simulink model "Simulation_FL_BB"  (R2023a)
settings: Solver=VariableStepAuto  StartTime=0.0  StopTime=50  RelTol=1e-3
settings Model: Creator=j.acevedom  LastModifiedBy=j.acevedom

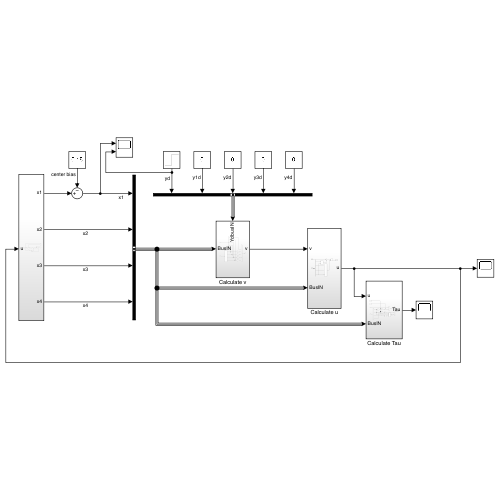
[thumbnail: Simulink's stored preview of the top-level diagram]
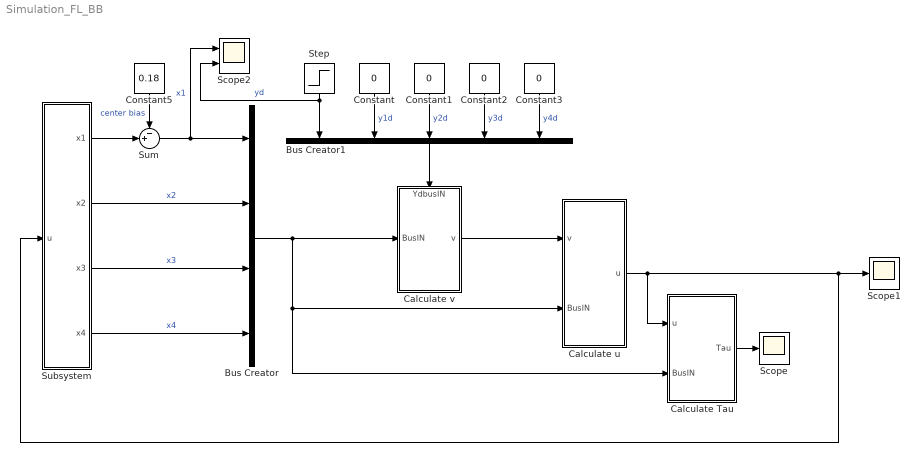
== system Simulation_FL_BB ==
  Bus Creator : BusCreator  Inputs=4
  Bus Creator1 : BusCreator  Inputs=5
  Calculate Tau : Subsystem
  Calculate u : Subsystem
  Calculate v : Subsystem
      settings: PortSchema="{\"entries\":[{\"content\":{\"sides\":[{\"content\":{\"connectorIds\":[\"In1\"]},\"type\":\"ConnectorPlacement.EquallySpacedRectSide\",\"uuid\":\"7c28e410-4806-4a94-8ccf-a14e347b0b8c\"},{\"content\":{\"connectorIds\":[\"Out1\"],\"side\":\"RIGHT\"},\"type\":\"ConnectorPlacement.EquallySpacedRectSide\",\"uuid\":\"f53d7206-bd2e-4f71-94df-5fcac3ff5314\"},{\"content\":{\"connectorIds\":[\"In2\"],\"side\":\"TOP\"},\"type\":\"ConnectorPlacement.EquallySpacedRectSide\",\"uuid\":\"6da5d2a6-a8d3-48a8-94f9-21942db04e1c\"}]},\"type\":\"ConnectorPlacement.EquallySpacedConnector\",\"uuid\":\"b4263dcd-b19e-4751-b906-56e55f698d2c\"}],\"packageUris\":[\"http://schema.mathworks.com/mf0/Connector/R2020b\"],\"version\":\"1.0\"}"
  Constant{,1..3} (4 alike) : Constant  Value=0
  Constant5 : Constant  Value=0.18
  Scope : Scope
  Scope1 : Scope
  Scope2 : Scope  NumInputPorts=2
  Step : Step  Time=10  After=0.1  SampleTime=0
  Subsystem : Subsystem
  Sum : Sum  Inputs=-+|
  wires:
  Calculate u/1(u) -> Scope1/1, Subsystem/1(u), Calculate Tau/1(u)
  Subsystem/3(x3) -> Bus Creator/3  "x3"
  Subsystem/4(x4) -> Bus Creator/4  "x4"
  Bus Creator/1 -> Calculate u/2(BusIN), Calculate Tau/2(BusIN), Calculate v/1(BusIN)
  Calculate v/1(v) -> Calculate u/1(v)
  Step/1 -> Scope2/2, Bus Creator1/1  "yd"
  Constant/1 -> Bus Creator1/2  "y1d"
  Constant1/1 -> Bus Creator1/3  "y2d"
  Constant2/1 -> Bus Creator1/4  "y3d"
  Constant3/1 -> Bus Creator1/5  "y4d"
  Bus Creator1/1 -> Calculate v/2(YdbusIN)
  Sum/1 -> Bus Creator/1, Scope2/1  "x1"
  Constant5/1 -> Sum/1  "center bias"
  Subsystem/2(x2) -> Bus Creator/2  "x2"
  Subsystem/1(x1) -> Sum/2
  Calculate Tau/1(Tau) -> Scope/1

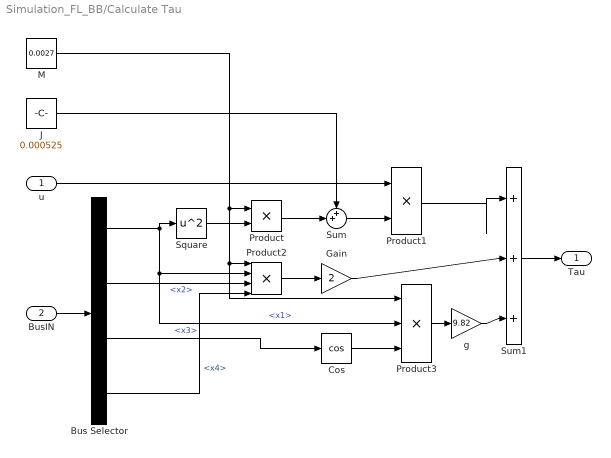
== system Simulation_FL_BB/Calculate Tau ==
  u : Inport
  BusIN : Inport  Port=2
  Bus Selector : BusSelector  OutputSignals=x1,x2,x3,x4
  Cos : Trigonometry  Operator=cos
  Gain : Gain  Gain=2
  J : Constant  Value=0.000525
  M : Constant  Value=0.0027
  Product : Product
  Product1 : Product
  Product2 : Product  Inputs=4
  Product3 : Product  Inputs=3
  Square : Math  Operator=square
  Sum : Sum  Inputs=++|
  Sum1 : Sum  Inputs=|+++
  g : Gain  Gain=9.82
  Tau : Outport
  wires:
  Square/1 -> Product/2
  M/1 -> Product2/1, Product3/1, Product/1
  Product/1 -> Sum/2
  J/1 -> Sum/1
  Sum/1 -> Product1/2
  u/1 -> Product1/1
  Bus Selector/4 -> Product2/4  "<x4>"
  Bus Selector/2 -> Product2/3  "<x2>"
  Bus Selector/1 -> Square/1, Product3/2, Product2/2  "<x1>"
  Product2/1 -> Gain/1
  Bus Selector/3 -> Cos/1  "<x3>"
  Product3/1 -> g/1
  Gain/1 -> Sum1/2
  Product1/1 -> Sum1/1
  Sum1/1 -> Tau/1
  BusIN/1 -> Bus Selector/1
  Cos/1 -> Product3/3
  g/1 -> Sum1/3

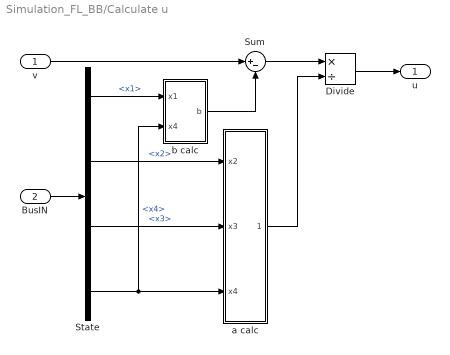
== system Simulation_FL_BB/Calculate u ==
  v : Inport
  BusIN : Inport  Port=2
  Divide : Product  Inputs=*/
  "State " : BusSelector  OutputSignals=x1,x2,x3,x4
  Sum : Sum  Inputs=|+-
  a calc : Subsystem
  b calc : Subsystem
  u : Outport
  wires:
  v/1 -> Sum/1
  Sum/1 -> Divide/1
  Divide/1 -> u/1
  "State "/4 -> b calc/2(x4), a calc/3(x4)  "<x4>"
  BusIN/1 -> "State "/1
  "State "/2 -> a calc/1(x2)  "<x2>"
  "State "/3 -> a calc/2(x3)  "<x3>"
  a calc/1(Out1) -> Divide/2
  "State "/1 -> b calc/1(x1)  "<x1>"
  b calc/1(b) -> Sum/2

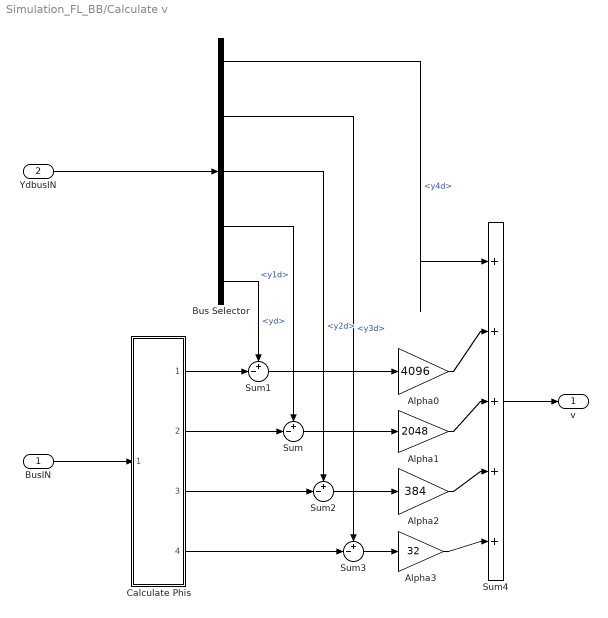
== system Simulation_FL_BB/Calculate v ==
  BusIN : Inport
  YdbusIN : Inport  Port=2
  Alpha0 : Gain  Gain=4096
  Alpha1 : Gain  Gain=2048
  Alpha2 : Gain  Gain=384
  Alpha3 : Gain  Gain=32
  Bus Selector : BusSelector  OutputSignals=y4d,y3d,y2d,y1d,yd
  Calculate Phis : Subsystem
  Sum{,1..3} (4 alike) : Sum  Inputs=+-|
  Sum4 : Sum  Inputs=|+++++
  v : Outport
  wires:
  Sum2/1 -> Alpha2/1
  Sum3/1 -> Alpha3/1
  Bus Selector/5 -> Sum1/1  "<yd>"
  Calculate Phis/1(Phi1) -> Sum1/2
  Bus Selector/1 -> Sum4/1  "<y4d>"
  Bus Selector/2 -> Sum3/1  "<y3d>"
  Bus Selector/3 -> Sum2/1  "<y2d>"
  Alpha1/1 -> Sum4/3
  Alpha0/1 -> Sum4/2
  Alpha2/1 -> Sum4/4
  Sum/1 -> Alpha1/1
  Bus Selector/4 -> Sum/1  "<y1d>"
  Alpha3/1 -> Sum4/5
  Calculate Phis/4(phi4) -> Sum3/2
  Sum1/1 -> Alpha0/1
  Calculate Phis/2(Phi2) -> Sum/2
  Calculate Phis/3(phi3) -> Sum2/2
  BusIN/1 -> Calculate Phis/1(BusIN)
  Sum4/1 -> v/1
  YdbusIN/1 -> Bus Selector/1

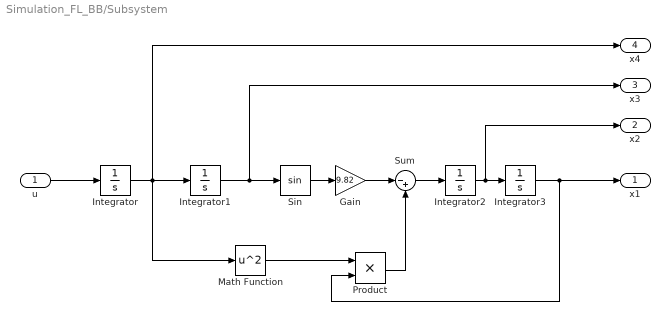
== system Simulation_FL_BB/Subsystem ==
  u : Inport
  Gain : Gain  Gain=9.82
  Integrator{,1..3} (4 alike) : Integrator
  Math Function : Math  Operator=square
  Product : Product
  Sin : Trigonometry
  Sum : Sum  Inputs=|-+
  x1 : Outport
  x2 : Outport  Port=2
  x3 : Outport  Port=3
  x4 : Outport  Port=4
  wires:
  u/1 -> Integrator/1
  Integrator/1 -> x4/1, Math Function/1, Integrator1/1
  Integrator1/1 -> Sin/1, x3/1
  Integrator2/1 -> x2/1, Integrator3/1
  Integrator3/1 -> x1/1, Product/2
  Math Function/1 -> Product/1
  Sum/1 -> Integrator2/1
  Product/1 -> Sum/2
  Gain/1 -> Sum/1
  Sin/1 -> Gain/1

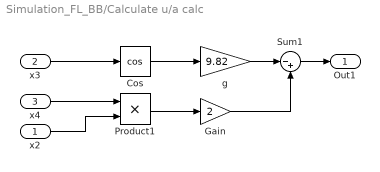
== system Simulation_FL_BB/Calculate u/a calc ==
  x2 : Inport
  x3 : Inport  Port=2
  x4 : Inport  Port=3
  Cos : Trigonometry  Operator=cos
  Gain : Gain  Gain=2
  Product1 : Product
  Sum1 : Sum  Inputs=|-+
  g : Gain  Gain=9.82
  Out1 : Outport
  wires:
  Product1/1 -> Gain/1
  Sum1/1 -> Out1/1
  Gain/1 -> Sum1/2
  Cos/1 -> g/1
  g/1 -> Sum1/1
  x3/1 -> Cos/1
  x4/1 -> Product1/1
  x2/1 -> Product1/2

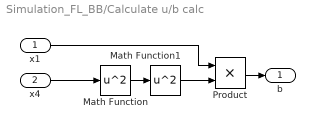
== system Simulation_FL_BB/Calculate u/b calc ==
  x1 : Inport
  x4 : Inport  Port=2
  Math Function : Math  Operator=square
  Math Function1 : Math  Operator=square
  Product : Product
  b : Outport
  wires:
  Math Function/1 -> Math Function1/1
  Math Function1/1 -> Product/2
  x1/1 -> Product/1
  x4/1 -> Math Function/1
  Product/1 -> b/1

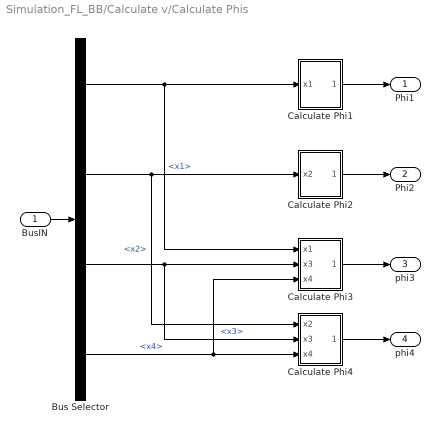
== system Simulation_FL_BB/Calculate v/Calculate Phis ==
  BusIN : Inport
  Bus Selector : BusSelector  OutputSignals=x1,x2,x3,x4
  Calculate Phi1 : Subsystem
  Calculate Phi2 : Subsystem
  Calculate Phi3 : Subsystem
  Calculate Phi4 : Subsystem
  Phi1 : Outport
  Phi2 : Outport  Port=2
  phi3 : Outport  Port=3
  phi4 : Outport  Port=4
  wires:
  Calculate Phi1/1(Phi1) -> Phi1/1
  Calculate Phi3/1(phi3) -> phi3/1
  BusIN/1 -> Bus Selector/1
  Calculate Phi4/1(phi4) -> phi4/1
  Calculate Phi2/1(Phi2) -> Phi2/1
  Bus Selector/1 -> Calculate Phi3/1(x1), Calculate Phi1/1(x1)  "<x1>"
  Bus Selector/2 -> Calculate Phi4/1(x2), Calculate Phi2/1(x2)  "<x2>"
  Bus Selector/3 -> Calculate Phi4/2(x3), Calculate Phi3/2(x3)  "<x3>"
  Bus Selector/4 -> Calculate Phi4/3(x4), Calculate Phi3/3(x4)  "<x4>"

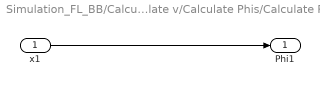
== system Simulation_FL_BB/Calculate v/Calculate Phis/Calculate Phi1 ==
  x1 : Inport
  Phi1 : Outport
  wires:
  x1/1 -> Phi1/1

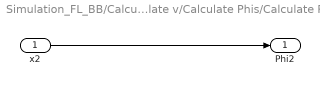
== system Simulation_FL_BB/Calculate v/Calculate Phis/Calculate Phi2 ==
  x2 : Inport
  Phi2 : Outport
  wires:
  x2/1 -> Phi2/1

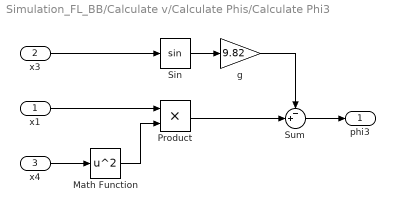
== system Simulation_FL_BB/Calculate v/Calculate Phis/Calculate Phi3 ==
  x1 : Inport
  x3 : Inport  Port=2
  x4 : Inport  Port=3
  Math Function : Math  Operator=square
  Product : Product
  Sin : Trigonometry
  Sum : Sum  Inputs=-+|
  g : Gain  Gain=9.82
  phi3 : Outport
  wires:
  x4/1 -> Math Function/1
  x1/1 -> Product/1
  Math Function/1 -> Product/2
  x3/1 -> Sin/1
  Product/1 -> Sum/2
  g/1 -> Sum/1
  Sum/1 -> phi3/1
  Sin/1 -> g/1

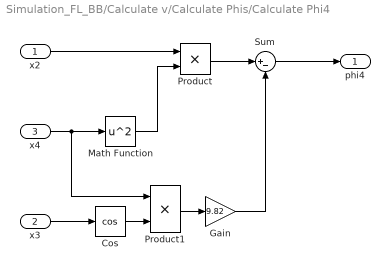
== system Simulation_FL_BB/Calculate v/Calculate Phis/Calculate Phi4 ==
  x2 : Inport
  x3 : Inport  Port=2
  x4 : Inport  Port=3
  Cos : Trigonometry  Operator=cos
  Gain : Gain  Gain=9.82
  Math Function : Math  Operator=square
  Product : Product
  Product1 : Product
  Sum : Sum  Inputs=|+-
  phi4 : Outport
  wires:
  x4/1 -> Product1/1, Math Function/1
  x2/1 -> Product/1
  Math Function/1 -> Product/2
  x3/1 -> Cos/1
  Product1/1 -> Gain/1
  Product/1 -> Sum/1
  Sum/1 -> phi4/1
  Cos/1 -> Product1/2
  Gain/1 -> Sum/2
